simulink model "simulationDCMotor"  (R2025b)
settings: Solver=VariableStepAuto  StartTime=0.0  StopTime=600  RelTol=1e-3
values from neighbouring files (symbols this model uses):
  kp = 1000    [DCMotor.m]
  Td = 0.5    [DCMotor.m]
  theta_ref = 1    [DCMotor.m]
  Ti = 1    [DCMotor.m]
undefined symbols (not defined in the file or in its folder): G_den, G_num
settings Model: Creator=Facundo  LastModifiedBy=Facundo

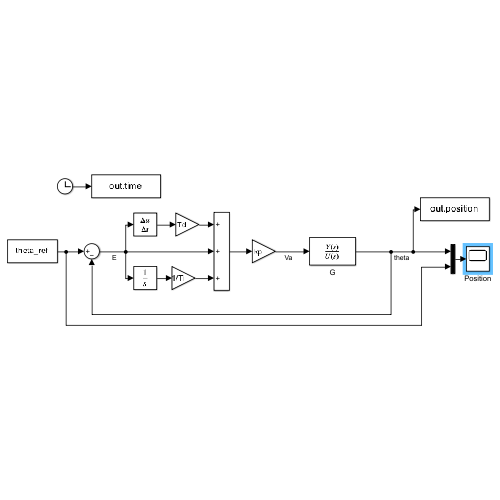
[thumbnail: Simulink's stored preview of the top-level diagram]
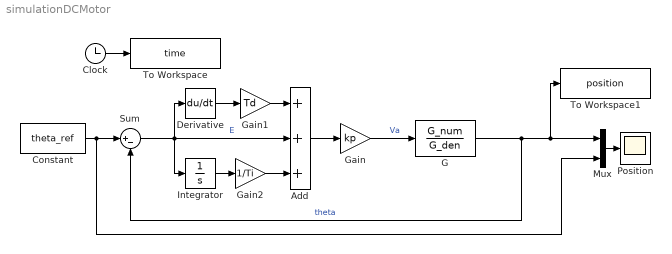
== system simulationDCMotor ==
  Add : Sum  Inputs=+++
  Clock : Clock
  Constant : Constant  Value=theta_ref
  Derivative : Derivative
  G : TransferFcn  Numerator=G_num  Denominator=G_den
  Gain : Gain  Gain=kp
  Gain1 : Gain  Gain=Td
  Gain2 : Gain  Gain=1/Ti
  Integrator : Integrator
  Mux : Mux  Inputs=2
  Position : Scope
      settings: ActiveDisplayYMinimum=-0.0033003300330032292  ActiveDisplayYMaximum=1.0218646864686469
  Sum : Sum  Inputs=|+-
  To Workspace : ToWorkspace  VariableName=time  SaveFormat=Timeseries  SampleTime=-1
  To Workspace1 : ToWorkspace  VariableName=position  SaveFormat=Timeseries  SampleTime=-1
  wires:
  Clock/1 -> To Workspace/1
  Constant/1 -> Mux/2, Sum/1
  G/1 -> Sum/2, Mux/1, To Workspace1/1  "theta"
  Sum/1 -> Integrator/1, Derivative/1, Add/2  "E"
  Add/1 -> Gain/1
  Gain/1 -> G/1  "Va"
  Derivative/1 -> Gain1/1
  Gain1/1 -> Add/1
  Integrator/1 -> Gain2/1
  Gain2/1 -> Add/3
  Mux/1 -> Position/1
